simulink model "MotorXploer"  (R2025b)
settings: Solver=FixedStepAuto  StartTime=0.0  StopTime=260  FixedStep=0.0005  RelTol=1e-3
undefined symbols (not defined in the file or in its folder): Blocking, LF, Non
libraries: amg_usbconverter_n_connect_lib x3, dspstat3 x1, eeStairGenerator x1
settings Model: Creator=beamk  LastModifiedBy=Asus

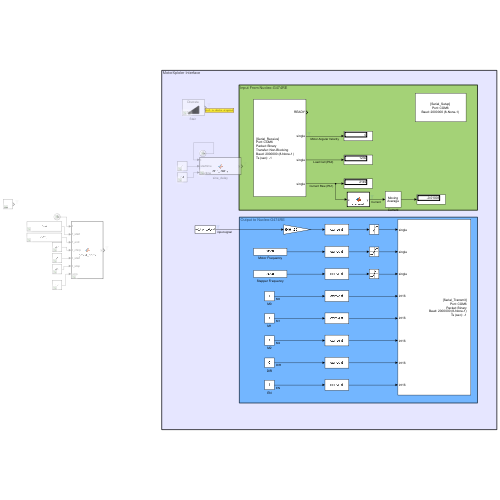
[thumbnail: Simulink's stored preview of the top-level diagram]
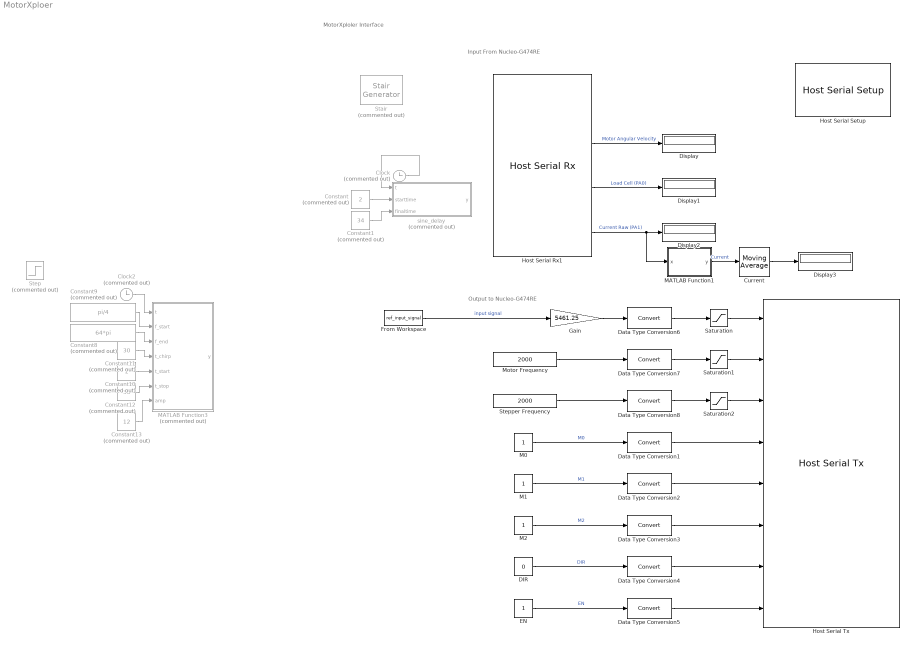
== system MotorXploer ==
  note: Output to Nucleo-G474RE
  note: Input From Nucleo-G474RE
  note: MotorXploler Interface
  Clock : Clock  Commented=on
  Clock2 : Clock  Commented=on
  Constant : Constant  Commented=on  Value=2
  Constant1 : Constant  Commented=on  Value=34
  Constant10 : Constant  Commented=on  Value=2
  Constant11 : Constant  Commented=on  Value=30
  Constant12 : Constant  Commented=on  Value=36
  Constant13 : Constant  Commented=on  Value=12
  Constant8 : Constant  Commented=on  Value=64*pi
  Constant9 : Constant  Commented=on  Value=pi/4
  Current : dspstat3/Moving Average  Method=Sliding window  ForgettingFactorPort=off  SpecifyWindowLength=on  WindowLength=500  OverlapLength=499  AllowArbitraryInputLength=off  ForgettingFactor=0.9  SimulateUsing=Interpreted execution
  DIR : Constant  Value=0
  Data Type Conversion{1..8} (8 alike) : DataTypeConversion  SaturateOnIntegerOverflow=off  RndMeth=Floor
  Display{,1..3} (4 alike) : Display
  EN : Constant
  From Workspace : FromWorkspace  VariableName=ref_input_signal
  Gain : Gain  Gain=5461.25
  Host Serial Rx1 : amg_usbconverter_n_connect_lib/Host Serial Rx  conf=rx  port=<auto>  baudrate=2000000  databits=8  parity=None  stopbit=1  flowcontrol=None  transfer=Non-Blocking  timeout=5  packetmode=Binary  enableinitialvalues=off  initialvalues=[]  binheader='25'  binterminator='4E'  porttype_double=0  porttype_single=3  porttype_int8=0  porttype_uint8=0  porttype_int16=0  porttype_uint16=0  porttype_int32=0  porttype_uint32=0  asciiformat='%f,%f,%d,%d'  rx_asciiterminator="LF (0x0A - \"\\n\")"  tx_asciiterminator="CRLF (0x0D 0x0A - \"\\r\\n\")"  sampletime=-1  enablecustomportlabel=off  cinputportlabel=0  coutputportlabel=A  portpinstr=0  blockid=HostSerialRx1  inputporttype=[]  inputportwidth=[]  inputportlabel={}  outputporttype=[3 1 1 1]  outputportwidth=[1 1 1 1]  outputportlabel={'READY','single','single','single'}  compat=0  optionstring=[]  autoport='COM6'
  Host Serial Setup : amg_usbconverter_n_connect_lib/Host Serial Setup  conf=setup  port=<auto>  baudrate=2000000  databits=8  parity=None  stopbit=1  flowcontrol=None  transfer=Blocking  timeout=2  packetmode=Binary  initialvalues=[]  binheader='7E 7E'  binterminator='03 03'  porttype_double=0  porttype_single=1  porttype_int8=0  porttype_uint8=0  porttype_int16=0  porttype_uint16=0  porttype_int32=0  porttype_uint32=2  asciiformat='%d %u %x'  rx_asciiterminator="CRLF (0x0D 0x0A - \"\\r\\n\")"  tx_asciiterminator="CRLF (0x0D 0x0A - \"\\r\\n\")"  sampletime=-1  enablecustomportlabel=off  cinputportlabel=0  coutputportlabel=A  portpinstr=0  blockid=HostSerialSetup  inputporttype=[]  inputportwidth=[]  inputportlabel={}  outputporttype=[]  outputportwidth=[]  outputportlabel={}  compat=0  optionstring=[]  autoport='COM6'
  Host Serial Tx : amg_usbconverter_n_connect_lib/Host Serial Tx  conf=tx  port=<auto>  baudrate=2000000  databits=8  parity=None  stopbit=1  flowcontrol=None  transfer=Blocking  timeout=2  packetmode=Binary  initialvalues=[]  binheader='25'  binterminator='4E'  porttype_double=0  porttype_single=3  porttype_int8=0  porttype_uint8=0  porttype_int16=5  porttype_uint16=0  porttype_int32=0  porttype_uint32=0  asciiformat='%d,%f'  rx_asciiterminator="CRLF (0x0D 0x0A - \"\\r\\n\")"  tx_asciiterminator="CRLF (0x0D 0x0A - \"\\r\\n\")"  sampletime=-1  enablecustomportlabel=off  cinputportlabel=0  coutputportlabel=A  portpinstr=0  blockid=HostSerialTx  inputporttype=[1 1 1 4 4 4 4 4]  inputportwidth=[1 1 1 1 1 1 1 1]  inputportlabel={'single','single','single','int16','int16','int16','int16','int16'}  outputporttype=[]  outputportwidth=[]  outputportlabel={}  compat=0  optionstring=[]  autoport='COM6'
      settings: SourceProductName=aMG USB Converter N
  M0 : Constant
  M1 : Constant
  M2 : Constant
  MATLAB Function1 : MATLAB Function  TreatAsAtomicUnit=on
  MATLAB Function3 : MATLAB Function  Commented=on  TreatAsAtomicUnit=on
  Motor Frequency : Constant  Value=2000  OutDataTypeStr=single
  Saturation : Saturate  UpperLimit=65535  LowerLimit=-65535
  Saturation1 : Saturate  UpperLimit=20000  LowerLimit=0
  Saturation2 : Saturate  UpperLimit=inf  LowerLimit=0
  "Stair " : eeStairGenerator/Stair Generator  Commented=on  LabelModeActiveChoice=Discrete  TimeInput=[2 4 6 8 10 12 14 16 18 20 22 24 26 28 30 32 34 36 38 40 42 44 46 48]  AmplitudeInput=[1 0 2 0 3 0 4 0 5 0 6 0 7 0 8 0 9 0 10 0 11 0 12 0]  SampleTime=0.0005  RepeatPattern=off  OutDataTypeStr=double
      settings: LibrarySourceBlock=ee_sl_lib/General Control/Stair Generator
  Step : Step  Commented=on  Time=2  After=12  SampleTime=0
  Stepper Frequency : Constant  Value=2000  OutDataTypeStr=single
  sine_delay : MATLAB Function  Commented=on  TreatAsAtomicUnit=on
  wires:
  Host Serial Rx1/2 -> Display/1  "Motor Angular Velocity"
  Host Serial Rx1/3 -> Display1/1  "Load Cell (PA0)"
  M0/1 -> Data Type Conversion1/1  "M0"
  EN/1 -> Data Type Conversion5/1  "EN"
  DIR/1 -> Data Type Conversion4/1  "DIR"
  M1/1 -> Data Type Conversion2/1  "M1"
  M2/1 -> Data Type Conversion3/1  "M2"
  Motor Frequency/1 -> Data Type Conversion7/1
  Stepper Frequency/1 -> Data Type Conversion8/1
  Data Type Conversion1/1 -> Host Serial Tx/4
  Data Type Conversion2/1 -> Host Serial Tx/5
  Data Type Conversion3/1 -> Host Serial Tx/6
  Data Type Conversion4/1 -> Host Serial Tx/7
  Data Type Conversion5/1 -> Host Serial Tx/8
  Data Type Conversion6/1 -> Saturation/1
  Saturation/1 -> Host Serial Tx/1
  Data Type Conversion7/1 -> Saturation1/1
  Data Type Conversion8/1 -> Saturation2/1
  Saturation1/1 -> Host Serial Tx/2
  Saturation2/1 -> Host Serial Tx/3
  Host Serial Rx1/4 -> MATLAB Function1/1(x), Display2/1  "Current Raw (PA1)"
  Current/1 -> Display3/1
  Constant8/1 -> MATLAB Function3/3(f_end)
  Constant13/1 -> MATLAB Function3/7(amp)
  Constant12/1 -> MATLAB Function3/6(t_stop)
  Clock2/1 -> MATLAB Function3/1(t)
  Constant10/1 -> MATLAB Function3/5(t_start)
  Constant11/1 -> MATLAB Function3/4(t_chirp)
  Constant9/1 -> MATLAB Function3/2(f_start)
  MATLAB Function1/1(y) -> Current/1  "Current"
  Gain/1 -> Data Type Conversion6/1
  Clock/1 -> sine_delay/1(t)
  Constant/1 -> sine_delay/2(starttime)
  Constant1/1 -> sine_delay/3(finaltime)
  From Workspace/1 -> Gain/1  "input signal"

== matlab function MotorXploer/MATLAB Function1 ==
  data: x input; y output
function y = convent(x)
    y = x;
    if x ~= 0
        y = -(0.0146 * x - 31.3702);
    end
end

== matlab function MotorXploer/sine_delay ==
  data: t input; y output; starttime input; finaltime input
function y = sine_delay(t, starttime, finaltime)

Amplitude = 12;
Freq = 2*pi;

if starttime < t && t < finaltime
    y = sin((t - starttime) * Freq) * Amplitude; 
elseif t >= finaltime
    y = sin((finaltime- starttime) * Freq) * Amplitude; 
else
    y=0;
end

== matlab function MotorXploer/MATLAB Function3 ==
  data: t input; y output; f_start input; f_end input; t_chirp input; t_start input; t_stop input; amp input
function y = gated_chirp(t, f_start, f_end, t_chirp, ...
                          t_start, t_stop, amp)
% t        : เวลาปัจจุบัน (วินาที)
% f_start  : ความถี่เริ่มต้น (Hz)
% f_end    : ความถี่สุดท้าย (Hz)
% t_chirp  : ระยะเวลา chirp (วินาที)
% t_start  : เวลาเริ่มสร้างสัญญาณ (วินาที)
% t_stop   : เวลาหยุดสัญญาณ (วินาที)
% amp      : แอมพลิจูด

y = 0;  % ค่าเริ่มต้นนอกช่วงเวลา

if (t >= t_start) && (t <= t_stop)

    % เวลาอ้างอิงภายใน chirp
    tau = t - t_start;

    % จำกัดไม่ให้เกินช่วง chirp
    if tau <= t_chirp
        % linear chirp
        k = (f_end - f_start) / t_chirp;   % sweep rate
        phase = ( f_start*tau + 0.5*k*tau^2 );
        y = amp * sin(phase);
    else
        y = 0;
    end
end
end
